simulink model "simulationBicineta"  (R2024a)
settings: Solver=VariableStepAuto  StartTime=0.0  StopTime=4860  RelTol=1e-3
settings DataIOCC: ExternalInput=[t, x1]

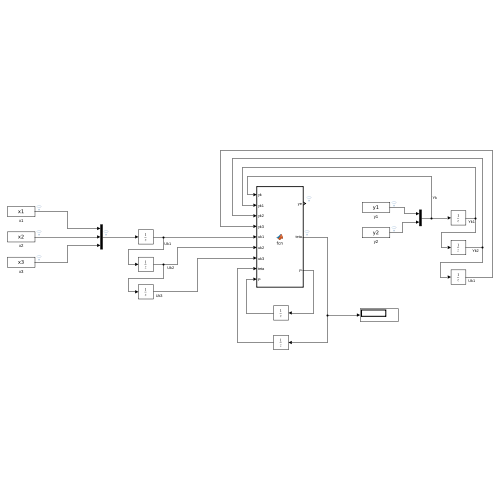
[thumbnail: Simulink's stored preview of the top-level diagram]
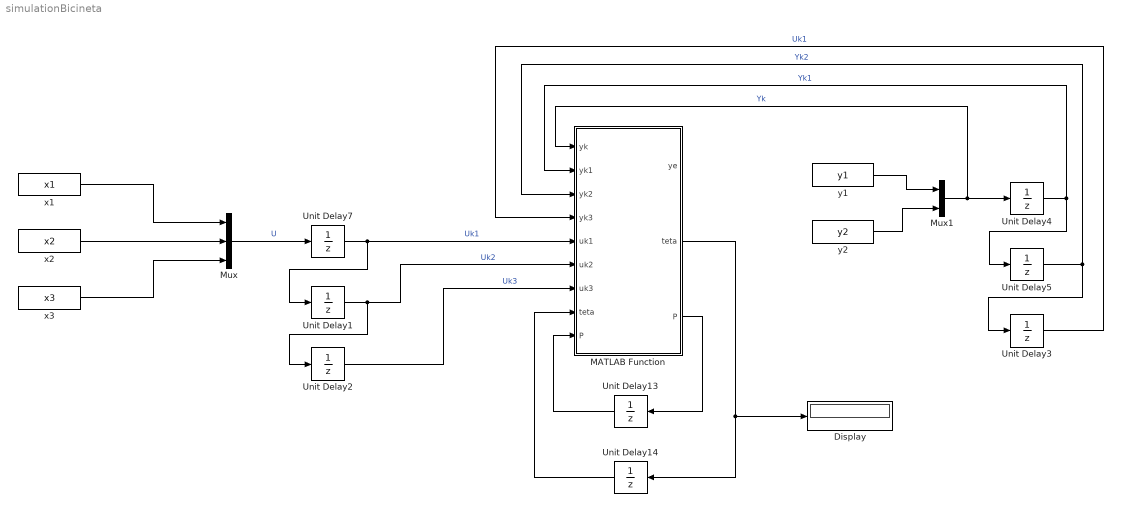
== system simulationBicineta ==
  Display : Display
  MATLAB Function : MATLAB Function  TreatAsAtomicUnit=on
  Mux : Mux  Inputs=3
  Mux1 : Mux  Inputs=2
  Unit Delay{1..5,7} (6 alike) : UnitDelay  SampleTime=-1  HasFrameUpgradeWarning=on
  Unit Delay13 : UnitDelay  InitialCondition=15000000000000000000000000*eye(15)  SampleTime=-1  HasFrameUpgradeWarning=on
  Unit Delay14 : UnitDelay  InitialCondition=zeros(15,2)  SampleTime=-1  HasFrameUpgradeWarning=on
  x1 : FromWorkspace  VariableName=x1  SampleTime=1.4853
  x2 : FromWorkspace  VariableName=x2  SampleTime=1.4853
  x3 : FromWorkspace  VariableName=x3  SampleTime=1.4853
  y1 : FromWorkspace  VariableName=y1  SampleTime=1.4853
  y2 : FromWorkspace  VariableName=y2  SampleTime=1.4853
  wires:
  MATLAB Function/3(P) -> Unit Delay13/1
  Unit Delay13/1 -> MATLAB Function/9("P ")
  Unit Delay14/1 -> MATLAB Function/8("teta ")
  MATLAB Function/2(teta) -> Unit Delay14/1, Display/1
  x2/1 -> Mux/2
  x1/1 -> Mux/1
  x3/1 -> Mux/3
  Mux/1 -> Unit Delay7/1  "U"
  Unit Delay7/1 -> Unit Delay1/1, MATLAB Function/5(uk1)  "Uk1"
  Unit Delay1/1 -> MATLAB Function/6(uk2), Unit Delay2/1  "Uk2"
  y2/1 -> Mux1/2
  y1/1 -> Mux1/1
  Mux1/1 -> Unit Delay4/1, MATLAB Function/1(yk)  "Yk"
  Unit Delay4/1 -> MATLAB Function/2(yk1), Unit Delay5/1  "Yk1"
  Unit Delay2/1 -> MATLAB Function/7(uk3)  "Uk3"
  Unit Delay5/1 -> Unit Delay3/1, MATLAB Function/3(yk2)  "Yk2"
  Unit Delay3/1 -> MATLAB Function/4(yk3)  "Uk1"

== matlab function simulationBicineta/MATLAB Function ==
  data: yk input; ye output; yk1 input; yk2 input; yk3 input; uk1 input; uk2 input; uk3 input; teta input; P input; teta output; P output
function [ye,teta,P] = fcn(yk,yk1,yk2,yk3,uk1,uk2,uk3,teta,P)


H=[-yk1,-yk2,-yk3,uk1,uk2,uk3]';
ye = H'*teta ;
teta=teta+P*H/(1+H'*P*H)*(yk-ye);
P=P-P*H/(H'*P*H+1)*H'*P;
